simulink model "needle"  (R2015a)
settings: Solver=ode5  StartTime=0.0  StopTime=10  FixedStep=0.01  RelTol=1e-3
libraries: simulink x2
settings Model: Creator=LAB425  LastModifiedBy=LAB425

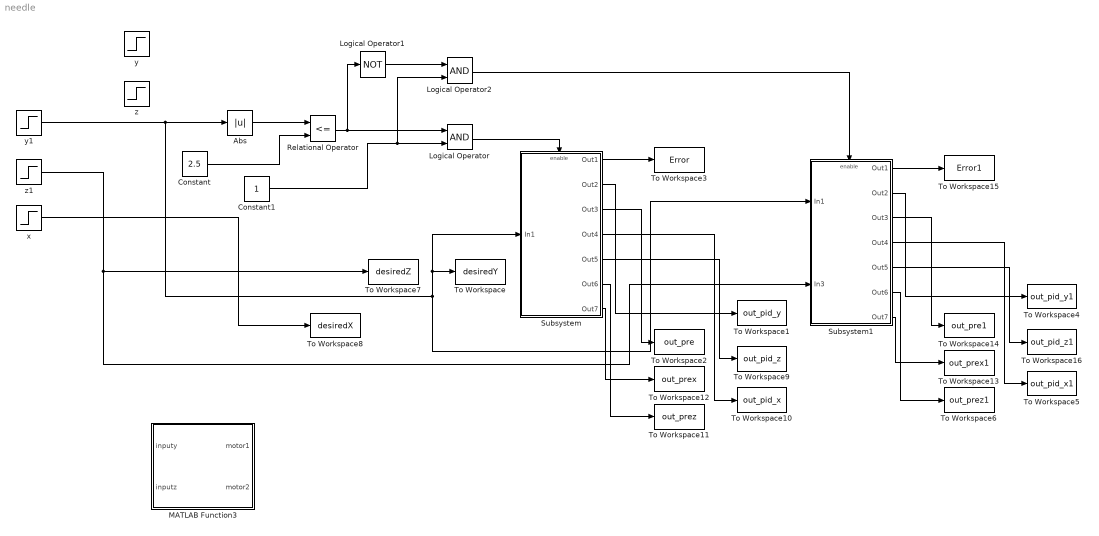
== system needle ==
  Abs : Abs
  Constant : Constant  Value=2.5
  Constant1 : Constant
  Logical Operator : Logic  AllPortsSameDT=off  OutDataTypeStr=boolean
  Logical Operator1 : Logic  Operator=NOT  AllPortsSameDT=off  OutDataTypeStr=boolean
  Logical Operator2 : Logic  AllPortsSameDT=off  OutDataTypeStr=boolean
  MATLAB Function3 : MATLAB Function  TreatAsAtomicUnit=on
  Relational Operator : RelationalOperator  Operator=<=  OutDataTypeStr=boolean
  Subsystem : Subsystem
  Subsystem1 : Subsystem
  To Workspace : ToWorkspace  VariableName=desiredY  SaveFormat=Timeseries  SampleTime=-1
  To Workspace1 : ToWorkspace  VariableName=out_pid_y  SaveFormat=Timeseries  SampleTime=-1
  To Workspace10 : ToWorkspace  VariableName=out_pid_x  SaveFormat=Timeseries  SampleTime=-1
  To Workspace11 : ToWorkspace  VariableName=out_prez  SaveFormat=Timeseries  SampleTime=-1
  To Workspace12 : ToWorkspace  VariableName=out_prex  SaveFormat=Timeseries  SampleTime=-1
  To Workspace13 : ToWorkspace  VariableName=out_prex1  SaveFormat=Timeseries  SampleTime=-1
  To Workspace14 : ToWorkspace  VariableName=out_pre1  SaveFormat=Timeseries  SampleTime=-1
  To Workspace15 : ToWorkspace  VariableName=Error1  SaveFormat=Timeseries  SampleTime=-1
  To Workspace16 : ToWorkspace  VariableName=out_pid_z1  SaveFormat=Timeseries  SampleTime=-1
  To Workspace2 : ToWorkspace  VariableName=out_pre  SaveFormat=Timeseries  SampleTime=-1
  To Workspace3 : ToWorkspace  VariableName=Error  SaveFormat=Timeseries  SampleTime=-1
  To Workspace4 : ToWorkspace  VariableName=out_pid_y1  SaveFormat=Timeseries  SampleTime=-1
  To Workspace5 : ToWorkspace  VariableName=out_pid_x1  SaveFormat=Timeseries  SampleTime=-1
  To Workspace6 : ToWorkspace  VariableName=out_prez1  SaveFormat=Timeseries  SampleTime=-1
  To Workspace7 : ToWorkspace  VariableName=desiredZ  SaveFormat=Timeseries  SampleTime=-1
  To Workspace8 : ToWorkspace  VariableName=desiredX  SaveFormat=Timeseries  SampleTime=-1
  To Workspace9 : ToWorkspace  VariableName=out_pid_z  SaveFormat=Timeseries  SampleTime=-1
  x : Step  After=0  SampleTime=0
  y : Step  Time=0.2  After=3.53  SampleTime=0
  y1 : Step  Time=0.2  After=2.32  SampleTime=0
  z : Step  Time=0.2  SampleTime=0
  z1 : Step  Time=0.2  After=5 - sqrt(5*5-2.32*2.32)  SampleTime=0
  wires:
  Abs/1 -> Relational Operator/1
  Constant/1 -> Relational Operator/2
  Relational Operator/1 -> Logical Operator/1, Logical Operator1/1
  Constant1/1 -> Logical Operator2/2, Logical Operator/2
  Subsystem/1(Out1) -> To Workspace3/1
  Logical Operator/1 -> Subsystem/Enable
  Logical Operator1/1 -> Logical Operator2/1
  Subsystem/2(Out2) -> To Workspace1/1
  z1/1 -> Subsystem1/2(In3), To Workspace7/1
  x/1 -> To Workspace8/1
  Subsystem/3(Out3) -> To Workspace2/1
  Subsystem/5(Out5) -> To Workspace9/1
  Subsystem/4(Out4) -> To Workspace10/1
  Subsystem/6(Out6) -> To Workspace11/1
  Subsystem/7(Out7) -> To Workspace12/1
  y1/1 -> Subsystem1/1(In1), Subsystem/1(In1), To Workspace/1, Abs/1
  Subsystem1/1(Out1) -> To Workspace15/1
  Logical Operator2/1 -> Subsystem1/Enable
  Subsystem1/2(Out2) -> To Workspace4/1
  Subsystem1/3(Out3) -> To Workspace14/1
  Subsystem1/5(Out5) -> To Workspace16/1
  Subsystem1/4(Out4) -> To Workspace5/1
  Subsystem1/6(Out6) -> To Workspace6/1
  Subsystem1/7(Out7) -> To Workspace13/1

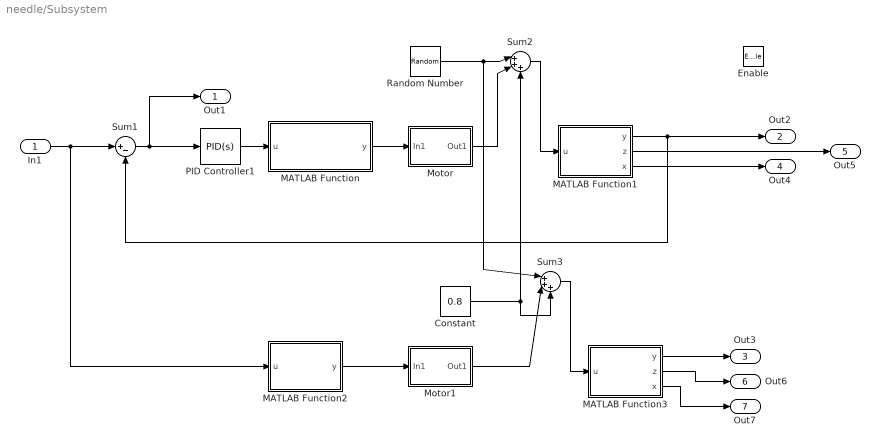
== system needle/Subsystem ==
  In1 : Inport
  Enable : EnablePort
  Constant : Constant  Value=0.8
  MATLAB Function : MATLAB Function  TreatAsAtomicUnit=on
  MATLAB Function1 : MATLAB Function  TreatAsAtomicUnit=on
  MATLAB Function2 : MATLAB Function  TreatAsAtomicUnit=on
  MATLAB Function3 : MATLAB Function  TreatAsAtomicUnit=on
  Motor : Subsystem
  Motor1 : Subsystem
  PID Controller1 : simulink/Continuous/PID Controller  Controller=PID  TimeDomain=Continuous-time  SampleTime=-1  IntegratorMethod=Forward Euler  FilterMethod=Forward Euler  Form=Parallel  UseFilter=on  ControllerParametersSource=internal  P=1.35  I=31  D=0  N=100  InitialConditionSource=internal  InitialConditionForIntegrator=0  InitialConditionForFilter=0  ExternalReset=none  LimitOutput=off  UpperSaturationLimit=inf  LowerSaturationLimit=-inf  LinearizeAsGain=on  AntiWindupMode=none  Kb=1  TrackingMode=off  Kt=1  PParamMin=[]  PParamMax=[]  IParamMin=[]  IParamMax=[]  DParamMin=[]  DParamMax=[]  NParamMin=[]  NParamMax=[]  KbParamMin=[]  KbParamMax=[]  KtParamMin=[]  KtParamMax=[]  POutMin=[]  POutMax=[]  IOutMin=[]  IOutMax=[]  DOutMin=[]  DOutMax=[]  NOutMin=[]  NOutMax=[]  KbOutMin=[]  KbOutMax=[]  KtOutMin=[]  KtOutMax=[]  IntegratorOutMin=[]  IntegratorOutMax=[]  FilterOutMin=[]  FilterOutMax=[]  SumOutMin=[]  SumOutMax=[]  SumI1OutMin=[]  SumI1OutMax=[]  SumI2OutMin=[]  SumI2OutMax=[]  SumI3OutMin=[]  SumI3OutMax=[]  SumDOutMin=[]  SumDOutMax=[]  SaturationOutMin=[]  SaturationOutMax=[]  IntegratorContinuousStateAttributes=''  IntegratorStateMustResolveToSignalObject=off  IntegratorRTWStateStorageClass=Auto  FilterContinuousStateAttributes=''  FilterStateMustResolveToSignalObject=off  FilterRTWStateStorageClass=Auto  DifferentiatorICPrevScaledInput=0  DifferentiatorOutMin=[]  DifferentiatorOutMax=[]
  Random Number : RandomNumber  Variance=0.01  Seed=1  SampleTime=0.01
  Sum1 : Sum  Inputs=|+-
  Sum2 : Sum  Inputs=|+++
  Sum3 : Sum  Inputs=|+++
  Out1 : Outport
  Out2 : Outport  Port=2
  Out3 : Outport  Port=3
  Out4 : Outport  Port=4
  Out5 : Outport  Port=5
  Out6 : Outport  Port=6
  Out7 : Outport  Port=7
  wires:
  Sum3/1 -> MATLAB Function3/1(u)
  Motor1/1(Out1) -> Sum3/2
  Random Number/1 -> Sum3/1, Sum2/1
  MATLAB Function3/1(y) -> Out3/1
  MATLAB Function2/1(y) -> Motor1/1(In1)
  MATLAB Function/1(y) -> Motor/1(In1)
  Sum2/1 -> MATLAB Function1/1(u)
  PID Controller1/1 -> MATLAB Function/1(u)
  Motor/1(Out1) -> Sum2/2
  Sum1/1 -> PID Controller1/1, Out1/1
  MATLAB Function1/1(y) -> Sum1/2, Out2/1
  In1/1 -> MATLAB Function2/1(u), Sum1/1
  MATLAB Function1/3(x) -> Out4/1
  MATLAB Function1/2(z) -> Out5/1
  MATLAB Function3/2(z) -> Out6/1
  MATLAB Function3/3(x) -> Out7/1
  Constant/1 -> Sum2/3, Sum3/3

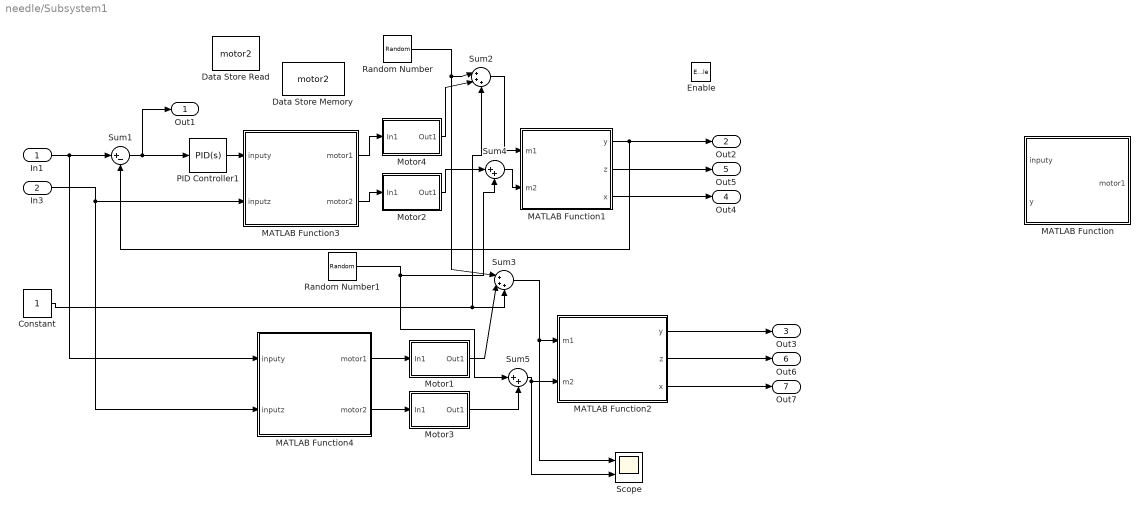
== system needle/Subsystem1 ==
  In1 : Inport
  In3 : Inport  Port=2
  Enable : EnablePort
  Constant : Constant
  Data Store Memory : DataStoreMemory  DataStoreName=motor2  ReadBeforeWriteMsg=warning  WriteAfterWriteMsg=warning  WriteAfterReadMsg=warning  OutDataTypeStr=double
  Data Store Read : DataStoreRead  DataStoreName=motor2
  MATLAB Function : MATLAB Function  TreatAsAtomicUnit=on
  MATLAB Function1 : MATLAB Function  TreatAsAtomicUnit=on
  MATLAB Function2 : MATLAB Function  TreatAsAtomicUnit=on
  MATLAB Function3 : MATLAB Function  TreatAsAtomicUnit=on
  MATLAB Function4 : MATLAB Function  TreatAsAtomicUnit=on
  Motor1 : Subsystem
  Motor2 : Subsystem
  Motor3 : Subsystem
  Motor4 : Subsystem
  PID Controller1 : simulink/Continuous/PID Controller  Controller=PID  TimeDomain=Continuous-time  SampleTime=-1  IntegratorMethod=Forward Euler  FilterMethod=Forward Euler  Form=Parallel  UseFilter=on  ControllerParametersSource=internal  P=1.3  I=20  D=0  N=100  InitialConditionSource=internal  InitialConditionForIntegrator=0  InitialConditionForFilter=0  ExternalReset=none  LimitOutput=off  UpperSaturationLimit=inf  LowerSaturationLimit=-inf  LinearizeAsGain=on  AntiWindupMode=none  Kb=1  TrackingMode=off  Kt=1  PParamMin=[]  PParamMax=[]  IParamMin=[]  IParamMax=[]  DParamMin=[]  DParamMax=[]  NParamMin=[]  NParamMax=[]  KbParamMin=[]  KbParamMax=[]  KtParamMin=[]  KtParamMax=[]  POutMin=[]  POutMax=[]  IOutMin=[]  IOutMax=[]  DOutMin=[]  DOutMax=[]  NOutMin=[]  NOutMax=[]  KbOutMin=[]  KbOutMax=[]  KtOutMin=[]  KtOutMax=[]  IntegratorOutMin=[]  IntegratorOutMax=[]  FilterOutMin=[]  FilterOutMax=[]  SumOutMin=[]  SumOutMax=[]  SumI1OutMin=[]  SumI1OutMax=[]  SumI2OutMin=[]  SumI2OutMax=[]  SumI3OutMin=[]  SumI3OutMax=[]  SumDOutMin=[]  SumDOutMax=[]  SaturationOutMin=[]  SaturationOutMax=[]  IntegratorContinuousStateAttributes=''  IntegratorStateMustResolveToSignalObject=off  IntegratorRTWStateStorageClass=Auto  FilterContinuousStateAttributes=''  FilterStateMustResolveToSignalObject=off  FilterRTWStateStorageClass=Auto  DifferentiatorICPrevScaledInput=0  DifferentiatorOutMin=[]  DifferentiatorOutMax=[]
  Random Number : RandomNumber  Variance=0.005  Seed=1  SampleTime=0.01
  Random Number1 : RandomNumber  Variance=0.005  Seed=1  SampleTime=0.01
  Scope : Scope  NumInputPorts=2
      settings: YMin=-5~-5  YMax=5~5
  Sum1 : Sum  Inputs=|+-
  Sum2 : Sum  Inputs=|+++
  Sum3 : Sum  Inputs=|+++
  Sum4 : Sum  Inputs=|++
  Sum5 : Sum  Inputs=|++
  Out1 : Outport
  Out2 : Outport  Port=2
  Out3 : Outport  Port=3
  Out4 : Outport  Port=4
  Out5 : Outport  Port=5
  Out6 : Outport  Port=6
  Out7 : Outport  Port=7
  wires:
  Sum3/1 -> Scope/1, MATLAB Function2/1(m1)
  Motor1/1(Out1) -> Sum3/2
  Random Number/1 -> Sum3/1, Sum2/1
  MATLAB Function2/1(y) -> Out3/1
  MATLAB Function4/1(motor1) -> Motor1/1(In1)
  Sum2/1 -> MATLAB Function1/1(m1)
  PID Controller1/1 -> MATLAB Function3/1(inputy)
  Sum1/1 -> PID Controller1/1, Out1/1
  MATLAB Function1/1(y) -> Sum1/2, Out2/1
  In1/1 -> MATLAB Function4/1(inputy), Sum1/1
  MATLAB Function1/3(x) -> Out4/1
  MATLAB Function1/2(z) -> Out5/1
  MATLAB Function2/2(z) -> Out6/1
  MATLAB Function2/3(x) -> Out7/1
  In3/1 -> MATLAB Function4/2(inputz), MATLAB Function3/2(inputz)
  MATLAB Function4/2(motor2) -> Motor3/1(In1)
  Random Number1/1 -> Sum5/1, Sum4/2
  Motor3/1(Out1) -> Sum5/2
  Sum5/1 -> Scope/2, MATLAB Function2/2(m2)
  MATLAB Function3/1(motor1) -> Motor4/1(In1)
  Motor4/1(Out1) -> Sum2/2
  Motor2/1(Out1) -> Sum4/1
  Sum4/1 -> MATLAB Function1/2(m2)
  Constant/1 -> Sum2/3, Sum3/3
  MATLAB Function3/2(motor2) -> Motor2/1(In1)

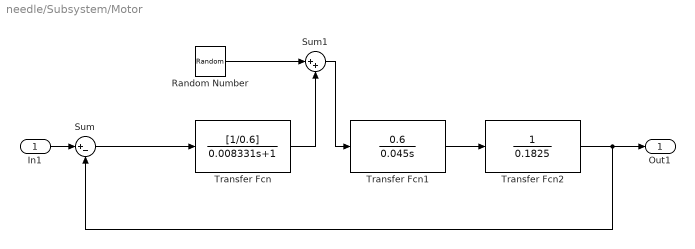
== system needle/Subsystem/Motor ==
  In1 : Inport
  Random Number : RandomNumber  Variance=0.1  SampleTime=0.01
  Sum : Sum  Inputs=|+-
  Sum1 : Sum  Inputs=|++
  Transfer Fcn : TransferFcn  Numerator=[1/0.6]  Denominator=[0.008331 1]
  Transfer Fcn1 : TransferFcn  Numerator=[0.6]  Denominator=[0.045 0]
  Transfer Fcn2 : TransferFcn  Denominator=[0.1825]
  Out1 : Outport
  wires:
  Transfer Fcn2/1 -> Sum/2, Out1/1
  Transfer Fcn1/1 -> Transfer Fcn2/1
  Sum1/1 -> Transfer Fcn1/1
  Random Number/1 -> Sum1/1
  Transfer Fcn/1 -> Sum1/2
  Sum/1 -> Transfer Fcn/1
  In1/1 -> Sum/1

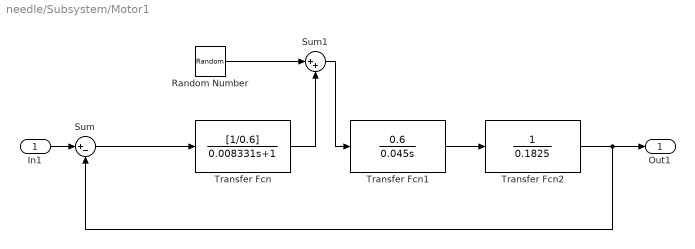
== system needle/Subsystem/Motor1 ==
  In1 : Inport
  Random Number : RandomNumber  Variance=0.1  SampleTime=0.01
  Sum : Sum  Inputs=|+-
  Sum1 : Sum  Inputs=|++
  Transfer Fcn : TransferFcn  Numerator=[1/0.6]  Denominator=[0.008331 1]
  Transfer Fcn1 : TransferFcn  Numerator=[0.6]  Denominator=[0.045 0]
  Transfer Fcn2 : TransferFcn  Denominator=[0.1825]
  Out1 : Outport
  wires:
  Transfer Fcn2/1 -> Sum/2, Out1/1
  Transfer Fcn1/1 -> Transfer Fcn2/1
  Sum1/1 -> Transfer Fcn1/1
  Random Number/1 -> Sum1/1
  Transfer Fcn/1 -> Sum1/2
  Sum/1 -> Transfer Fcn/1
  In1/1 -> Sum/1

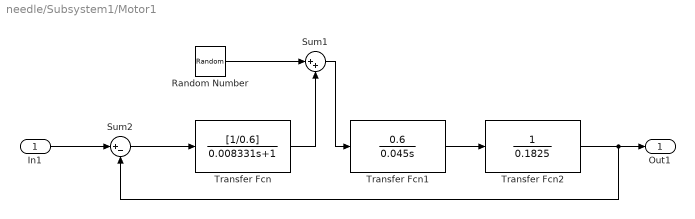
== system needle/Subsystem1/Motor1 ==
  In1 : Inport
  Random Number : RandomNumber  Variance=0.1  SampleTime=0.01
  Sum1 : Sum  Inputs=|++
  Sum2 : Sum  Inputs=|+-
  Transfer Fcn : TransferFcn  Numerator=[1/0.6]  Denominator=[0.008331 1]
  Transfer Fcn1 : TransferFcn  Numerator=[0.6]  Denominator=[0.045 0]
  Transfer Fcn2 : TransferFcn  Denominator=[0.1825]
  Out1 : Outport
  wires:
  Transfer Fcn2/1 -> Sum2/2, Out1/1
  Transfer Fcn1/1 -> Transfer Fcn2/1
  Sum1/1 -> Transfer Fcn1/1
  Random Number/1 -> Sum1/1
  Transfer Fcn/1 -> Sum1/2
  In1/1 -> Sum2/1
  Sum2/1 -> Transfer Fcn/1

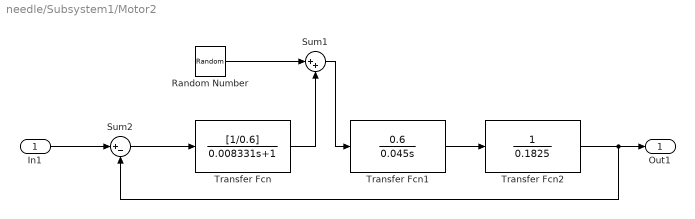
== system needle/Subsystem1/Motor2 ==
  In1 : Inport
  Random Number : RandomNumber  Variance=0.1  SampleTime=0.01
  Sum1 : Sum  Inputs=|++
  Sum2 : Sum  Inputs=|+-
  Transfer Fcn : TransferFcn  Numerator=[1/0.6]  Denominator=[0.008331 1]
  Transfer Fcn1 : TransferFcn  Numerator=[0.6]  Denominator=[0.045 0]
  Transfer Fcn2 : TransferFcn  Denominator=[0.1825]
  Out1 : Outport
  wires:
  Transfer Fcn2/1 -> Sum2/2, Out1/1
  Transfer Fcn1/1 -> Transfer Fcn2/1
  Sum1/1 -> Transfer Fcn1/1
  Random Number/1 -> Sum1/1
  Transfer Fcn/1 -> Sum1/2
  In1/1 -> Sum2/1
  Sum2/1 -> Transfer Fcn/1

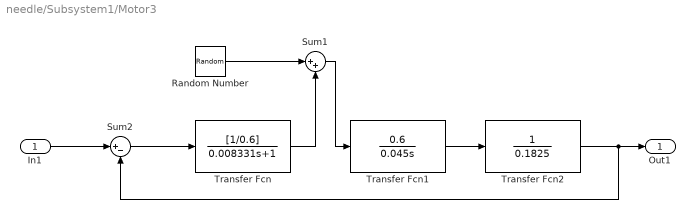
== system needle/Subsystem1/Motor3 ==
  In1 : Inport
  Random Number : RandomNumber  Variance=0.1  SampleTime=0.01
  Sum1 : Sum  Inputs=|++
  Sum2 : Sum  Inputs=|+-
  Transfer Fcn : TransferFcn  Numerator=[1/0.6]  Denominator=[0.008331 1]
  Transfer Fcn1 : TransferFcn  Numerator=[0.6]  Denominator=[0.045 0]
  Transfer Fcn2 : TransferFcn  Denominator=[0.1825]
  Out1 : Outport
  wires:
  Transfer Fcn2/1 -> Sum2/2, Out1/1
  Transfer Fcn1/1 -> Transfer Fcn2/1
  Sum1/1 -> Transfer Fcn1/1
  Random Number/1 -> Sum1/1
  Transfer Fcn/1 -> Sum1/2
  In1/1 -> Sum2/1
  Sum2/1 -> Transfer Fcn/1

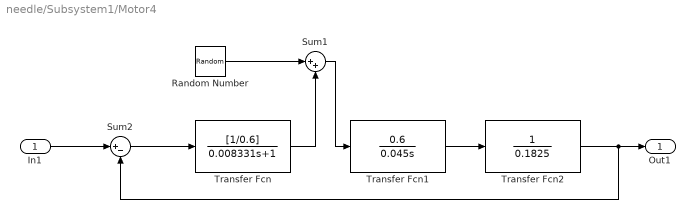
== system needle/Subsystem1/Motor4 ==
  In1 : Inport
  Random Number : RandomNumber  Variance=0.1  SampleTime=0.01
  Sum1 : Sum  Inputs=|++
  Sum2 : Sum  Inputs=|+-
  Transfer Fcn : TransferFcn  Numerator=[1/0.6]  Denominator=[0.008331 1]
  Transfer Fcn1 : TransferFcn  Numerator=[0.6]  Denominator=[0.045 0]
  Transfer Fcn2 : TransferFcn  Denominator=[0.1825]
  Out1 : Outport
  wires:
  Transfer Fcn2/1 -> Sum2/2, Out1/1
  Transfer Fcn1/1 -> Transfer Fcn2/1
  Sum1/1 -> Transfer Fcn1/1
  Random Number/1 -> Sum1/1
  Transfer Fcn/1 -> Sum1/2
  In1/1 -> Sum2/1
  Sum2/1 -> Transfer Fcn/1

== matlab function needle/Subsystem/MATLAB Function1 ==
  data: u input; y output; z output; x output
function [y,z,x] = forward(u)
%#codegen

% y = u;
% mid = asin(u/5);
% 
% mid2 = 3 * tan(mid);
% 
% ymid = mid2 / 0.2;
% 
% y = pi * ymid;

d = 0.2 * u / pi;

theta = atan2(d,3);

y = sin(theta) * 5;

x = 0;

z = 5 - sqrt(5^2 - y^2);

== matlab function needle/Subsystem/MATLAB Function ==
  data: u input; y output
function y = inv(u)
%#codegen
% u = 2.5
% y = u;
mid = asin(u/5);

mid2 = 3 * tan(mid);

ymid = mid2 / 0.2;

y = pi * ymid;

== matlab function needle/Subsystem/MATLAB Function2 ==
  data: u input; y output
function y = inv(u)
%#codegen

% y = u;
mid = asin(u/5);

mid2 = 3 * tan(mid);

ymid = mid2 / 0.2;

y = pi * ymid;

== matlab function needle/Subsystem/MATLAB Function3 ==
  data: u input; y output; z output; x output
function [y,z,x] = forward(u)
%#codegen

% y = u;
% mid = asin(u/5);
% 
% mid2 = 3 * tan(mid);
% 
% ymid = mid2 / 0.2;
% 
% y = pi * ymid;

d = 0.2 * u / pi;

theta = atan2(d,3);

y = sin(theta) * 5;

x = 0;

z = 5 - sqrt(5^2 - y^2);

== matlab function needle/Subsystem1/MATLAB Function ==
  data: inputy input; motor1 output; motor2 data_store_memory; y input
function motor1 = inv(inputy,y)
%#codegen
% u = 2.5
% y = u;
% ToDeg = 180 / pi;
% 
% ToRad = pi / 180;
global motor2

u = 2.5;

mid = asin(u/5);

mid2 = 3 * tan(mid);

ymid = mid2 / 0.2;

motor1 = pi * ymid;

% L = abs(mid2) + abs(inputy);

% ylow = sqrt(5^2 - (5 - inputz)^2);
% 
% yl = L - ylow;
% 
% motor2mid = yl / 0.2;
% 
% motor2 = motor2mid * pi;

if y >= 0
    if inputy > 0.1
        motor2 = motor2 + 0.4;
    elseif inputy < -0.1
        motor2 = motor2 - 1;
    end
else
    if inputy > 0.1
        motor2 = motor2 - 1;
    elseif inputy < -0.1
        motor2 = motor2 + 0.4;
    end
end

== matlab function needle/Subsystem1/MATLAB Function1 ==
  data: m1 input; y output; z output; x output; m2 input
function [y,z,x] = forward(m1,m2)
%#codegen

% y = u;
% mid = asin(u/5);
% 
% mid2 = 3 * tan(mid);
% 
% ymid = mid2 / 0.2;
% 
% y = pi * ymid;

d1 = 0.2 * m1 / pi;

d2 = 0.2 * m2 / pi;

D = d1 + d2;

theta = atan2(D,3);

x = 0;

% z = sqrt(5^2 + y^2);

y1 = 5 * sin(theta);

y = y1 + d2;

% z = 5 - 5 * cos(theta);

z = 5 - sqrt(5*5- y1*y1);

% z = d1;

== matlab function needle/Subsystem1/MATLAB Function2 ==
  data: m1 input; y output; z output; x output; m2 input
function [y,z,x] = forward(m1,m2)
%#codegen

% y = u;
% mid = asin(u/5);
% 
% mid2 = 3 * tan(mid);
% 
% ymid = mid2 / 0.2;
% 
% y = pi * ymid;

d1 = 0.2 * m1 / pi;

d2 = 0.2 * m2 / pi;

D = d1 + d2;

theta = atan2(D,3);

x = 0;

% z = sqrt(5^2 + y^2);

y1 = 5 * sin(theta);

y = abs(y1) + abs(d2);

z = 5 - 5 * cos(theta);

== matlab function needle/Subsystem1/MATLAB Function3 ==
  data: inputy input; motor1 output; inputz input; motor2 output
function [motor1,motor2] = inv(inputy,inputz)
%#codegen
% u = 2.5
% y = u;
% ToDeg = 180 / pi;
% 
% ToRad = pi / 180;

u = 2.5;

mid = asin(u/5);

mid2 = 3 * tan(mid);

ymid = mid2 / 0.2;%转动电机的总圈数

motor1 = pi * ymid;%圈数 × 2pi

X = 5 - inputz;

Y = sqrt(5^2 - X^2);

motor2move = inputy - Y;

motor2mid = motor2move / 0.2;

motor2 = pi * motor2mid;

== matlab function needle/Subsystem1/MATLAB Function4 ==
  data: inputy input; motor1 output; inputz input; motor2 output
function [motor1,motor2] = inv(inputy,inputz)
%#codegen
% u = 2.5
% y = u;
% ToDeg = 180 / pi;
% 
% ToRad = pi / 180;

u = 2.5;

mid = asin(u/5);

mid2 = 3 * tan(mid);

ymid = mid2 / 0.2;%转动电机的总圈数

motor1 = pi * ymid;%圈数 × 2pi

X = 5 - inputz;

Y = sqrt(5^2 - X^2);

motor2move = inputy - Y;

motor2mid = motor2move / 0.2;

motor2 = pi * motor2mid;

== matlab function needle/MATLAB Function3 ==
  data: inputy input; motor1 output; inputz input; motor2 output
function [motor1,motor2] = inv(inputy,inputz)
%#codegen
% u = 2.5
% y = u;
% ToDeg = 180 / pi;
% 
% ToRad = pi / 180;

u = 2.5;

mid = asin(u/5);

mid2 = 3 * tan(mid);

ymid = mid2 / 0.2;%转动电机的总圈数

motor1 = pi * ymid;%圈数 × 2pi

X = 5 - inputz;

Y = sqrt(5^2 - X^2);

motor2move = inputy - Y;

motor2mid = motor2move / 0.2;

motor2 = pi * motor2mid;
